simulink model "zerodyn"  (R2017b)
settings: Solver=VariableStepAuto  StartTime=0.0  StopTime=10.0  RelTol=1e-3
settings Model: Creator=exo-hand  LastModifiedBy=exo-hand

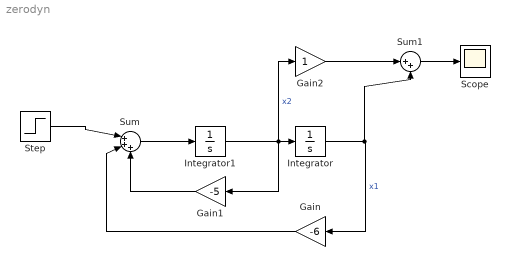
== system zerodyn ==
  Gain : Gain  Gain=-6
  Gain1 : Gain  Gain=-5
  Gain2 : Gain
  Integrator : Integrator
  Integrator1 : Integrator
  Scope : Scope
  Step : Step  SampleTime=0
  Sum : Sum  Inputs=|+++
  Sum1 : Sum  Inputs=|++
  wires:
  Integrator1/1 -> Gain2/1, Gain1/1, Integrator/1  "x2"
  Integrator/1 -> Sum1/2, Gain/1  "x1"
  Sum/1 -> Integrator1/1
  Gain1/1 -> Sum/3
  Gain/1 -> Sum/2
  Gain2/1 -> Sum1/1
  Step/1 -> Sum/1
  Sum1/1 -> Scope/1
